simulink model "on_off"  (R2022b)
settings: Solver=VariableStepAuto  StartTime=0.0  StopTime=inf  RelTol=1e-3
settings Model: Creator=rlawo  LastModifiedBy=user

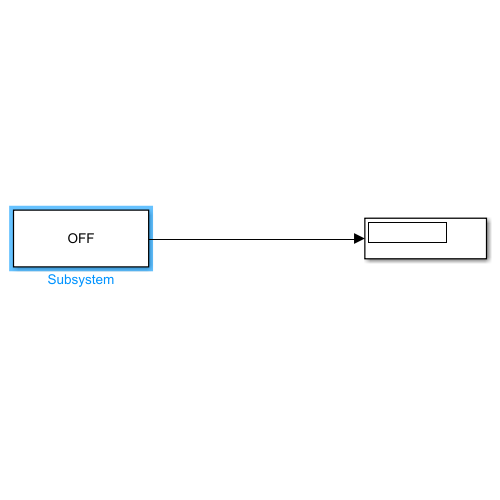
[thumbnail: Simulink's stored preview of the top-level diagram]
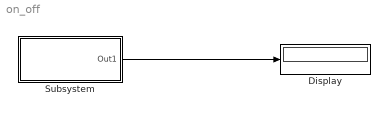
== system on_off ==
  Display : Display
  Subsystem : Subsystem  StartFcn=|  mask{str=OFF}
      | set_param(gcb, 'str', 'OFF');
      | set_param([gcb '/Constant'], 'Value', '0');
      mask prompts: str "Display name :"
      settings: OpenFcn=|
      | old_val = get_param([gcb '/Constant'], 'Value');
      | 
      | switch old_val
      | case '0'
      |     set_param(gcb, 'str', 'ON');
      |     set_param([gcb '/Constant'], 'Value', '1');
      | 
      | case '1'
      |     set_param(gcb, 'str', 'OFF');
      |     set_param([gcb '/Constant'], 'Value', '0');
      | 
      | otherwise
      |     set_param(gcb, 'str', 'OFF');
      |     set_param([gcb '/Constant'], 'Value', '0');
      | 
      | end
      mask DialogControl ParameterGroupVar Prompt: 파라미터
      mask Display: disp(get_param(gcb,'str'));
  wires:
  Subsystem/1(Out1) -> Display/1

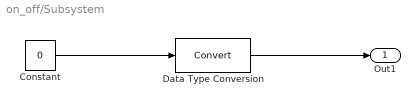
== system on_off/Subsystem ==
  Constant : Constant  Value=0
  "Data Type Conversion " : DataTypeConversion  SaturateOnIntegerOverflow=off  RndMeth=Floor
  Out1 : Outport
  wires:
  Constant/1 -> "Data Type Conversion "/1
  "Data Type Conversion "/1 -> Out1/1
